simulink model "PPS_EGO_State_Display"  (Simulink 7.6)
settings: Solver=FixedStepDiscrete  SolverMode=SingleTasking  StartTime=0.0  StopTime=inf  FixedStep=0.01  RelTol=1e-3
InitFcn:
  | global det_flag;
  | 
  | det_flag = 0;
libraries: simulink x1
settings Model: Creator=Krzysztof  LastModifiedBy=pastora
settings DataIOCC: LimitDataPoints=off  MaxDataPoints=1  SaveOutput=off  DSMLogging=off  InspectSignalLogs=on
settings OptimizationCC: InlineParams=on
settings DebuggingCC: UnknownTsInhSupMsg=none
settings ModelReferenceCC: ModelReferenceNumInstancesAllowed=Single

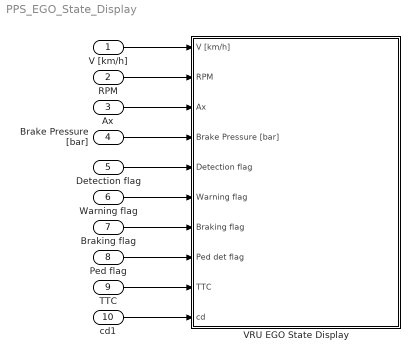
== system PPS_EGO_State_Display ==
  V [km/h] : Inport
  RPM : Inport  Port=2
  Ax : Inport  Port=3
  Brake Pressure [bar] : Inport  Port=4
  Detection flag : Inport  Port=5
  Warning flag : Inport  Port=6
  Braking flag : Inport  Port=7
  Ped flag : Inport  Port=8
  TTC : Inport  Port=9
  cd1 : Inport  Port=10
  VRU EGO State Display : Subsystem  mask{brakepressure=150, mfreq=100, dfreq=25}
      mask prompts: brakepressure "Maximum value of braking pressure [bar]"; mfreq "Model frequency [Hz]"; dfreq "Display frequency [Hz]"
  wires:
  V [km/h]/1 -> VRU EGO State Display/1(V [km/h])
  RPM/1 -> VRU EGO State Display/2(RPM)
  Brake Pressure [bar]/1 -> VRU EGO State Display/4(Brake Pressure [bar])
  Warning flag/1 -> VRU EGO State Display/6(Warning flag)
  Braking flag/1 -> VRU EGO State Display/7(Braking flag)
  Ped flag/1 -> VRU EGO State Display/8(Ped det flag)
  TTC/1 -> VRU EGO State Display/9(TTC)
  Detection flag/1 -> VRU EGO State Display/5(Detection flag)
  cd1/1 -> VRU EGO State Display/10(cd)
  Ax/1 -> VRU EGO State Display/3(Ax)

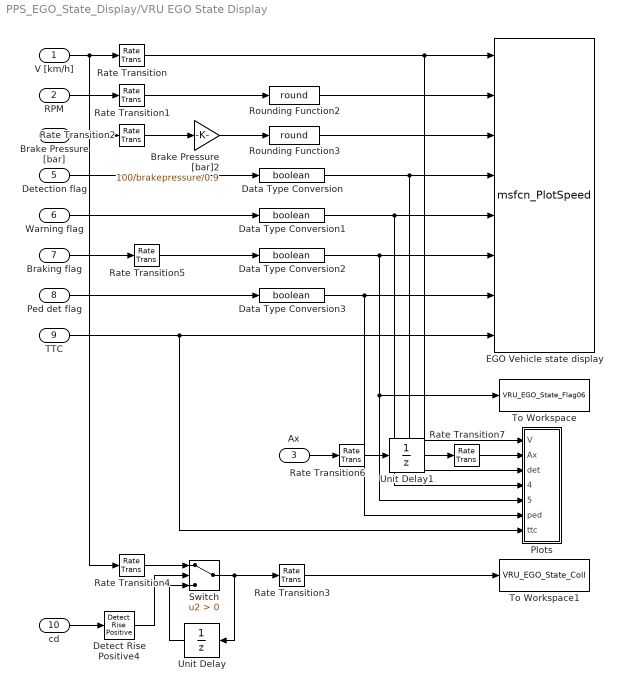
== system PPS_EGO_State_Display/VRU EGO State Display ==
  V [km/h] : Inport  SampleTime=[0,0]
  RPM : Inport  Port=2  SampleTime=[0,0]
  Ax : Inport  Port=3  SampleTime=[0,0]
  Brake Pressure [bar] : Inport  Port=4  SampleTime=[0,0]
  Detection flag : Inport  Port=5  OutDataTypeStr=boolean
  Warning flag : Inport  Port=6  OutDataTypeStr=boolean
  Braking flag : Inport  Port=7  OutDataTypeStr=boolean
  Ped det flag : Inport  Port=8  OutDataTypeStr=boolean
  TTC : Inport  Port=9  SampleTime=1/dfreq
  cd : Inport  Port=10  OutDataTypeStr=boolean  SampleTime=1/mfreq
  Brake Pressure [bar]2 : Gain  Gain=100/brakepressure/0.9
  Data Type Conversion{,1..3} (4 alike) : DataTypeConversion  OutDataTypeStr=boolean
  Detect Rise Positive4 : simulink/Logic and Bit Operations/Detect Rise Positive  SystemSampleTime=-1  vinit=0
  EGO Vehicle state display : M-S-Function  StopFcn=|  FunctionName=msfcn_PlotSpeed  Parameters=dfreq
      | CSpanel = findobj('Tag','cs_panel');                                                                                          
      | CSvalue = findobj('Tag','cs_value');                                                                                          
      | if VRU_EGO_State_Coll                                                                                                         
      |    % Collision occured                                                                                                        
      |    set(CSpanel, 'BorderWidth',2, 'ForegroundColor','Red', 'HighlightColor','Red', 'ShadowColor', 'Red');                      
      |    set(CSvalue, 'ForegroundColor','Red', 'String', strcat('Collision speed', sprintf( ' %.1f ',VRU_EGO_State_Coll), ' km/h'));
      |    set(CSpanel, 'Visible', 'On');                                                                                             
      |    set(CSvalue, 'Visible', 'On');                                                                                             
      | else                                                                                                                          
      |     if VRU_EGO_State_Flag06                                                                                                   
      |         % Collision almost occur                                                                                              
      | 	set(CSpanel, 'BorderWidth',2, 'ForegroundColor','Green', 'HighlightColor','Green', 'ShadowColor', 'Green');                  
      | 	set(CSvalue, 'ForegroundColor','Green', 'String', 'Collision avoided');                                                      
      |         set(CSpanel, 'Visible', 'On');                                                                                        
      |         set(CSvalue, 'Visible', 'On');                                                                                        
      |     else                                                                                                                      
      |         % No risk of collision                                                                                                
      | 	set(CSpanel, 'Visible', 'Off');                                                                                              
      |         set(CSvalue, 'Visible', 'Off');                                                                                       
      |     end                                                                                                                       
      | end                                                                                                                           
      | clear CSpanel CSvalue VRU_EGO_State_Flag06
  Plots : Subsystem  StopFcn=|
      | VRU_Speed_Profile(VRU_simout,VRU_EGO_State_Coll);
      | VRU_TTC_Profile(VRU_simout,VRU_EGO_State_Coll);
      mask Description:
      | The block calls functions:
      | * VRU_Speed_Profile
      | * VRU_TTC_Profile
      | to generate plots at the end of the simulation.
      | See stop callback of the block for more details.
  Rate Transition{,1..2,5,7} (5 alike) : RateTransition  Integrity=off  OutPortSampleTime=1/dfreq
  Rate Transition3 : RateTransition  Integrity=off  OutPortSampleTime=[0,0]
  Rate Transition4 : RateTransition  Integrity=off  OutPortSampleTime=1/mfreq
  Rate Transition6 : RateTransition  Integrity=off  OutPortSampleTimeOpt=Inherit  OutPortSampleTime=1/dfreq
  Rounding Function2 : Rounding  Operator=round
  Rounding Function3 : Rounding  Operator=round
  Switch : Switch  Criteria=u2 > Threshold  SampleTime=1/mfreq
  To Workspace : ToWorkspace  VariableName=VRU_EGO_State_Flag06  SampleTime=-1  SaveFormat=Array
      settings: MaxDataPoints=1
  To Workspace1 : ToWorkspace  VariableName=VRU_EGO_State_Coll  SampleTime=-1  SaveFormat=Array
      settings: MaxDataPoints=1
  Unit Delay : UnitDelay  SampleTime=1/mfreq
  Unit Delay1 : UnitDelay  SampleTime=-1
  wires:
  RPM/1 -> Rate Transition1/1
  Brake Pressure [bar]/1 -> Rate Transition2/1
  V [km/h]/1 -> Rate Transition/1, Rate Transition4/1
  Rounding Function2/1 -> EGO Vehicle state display/2
  Rounding Function3/1 -> EGO Vehicle state display/3
  Brake Pressure [bar]2/1 -> Rounding Function3/1
  Warning flag/1 -> Data Type Conversion1/1
  Ped det flag/1 -> Data Type Conversion3/1
  TTC/1 -> EGO Vehicle state display/8, Plots/7(ttc)
  Detection flag/1 -> Data Type Conversion/1
  Data Type Conversion/1 -> EGO Vehicle state display/4, Plots/3(det)
  Data Type Conversion1/1 -> EGO Vehicle state display/5, Plots/4(warn)
  Data Type Conversion2/1 -> EGO Vehicle state display/6, To Workspace/1, Plots/5(brake)
  Data Type Conversion3/1 -> EGO Vehicle state display/7, Plots/6(ped)
  Rate Transition/1 -> EGO Vehicle state display/1, Plots/1(V)
  Rate Transition1/1 -> Rounding Function2/1
  Rate Transition3/1 -> To Workspace1/1
  cd/1 -> Detect Rise Positive4/1
  Switch/1 -> Unit Delay/1, Rate Transition3/1
  Unit Delay/1 -> Switch/3
  Rate Transition4/1 -> Switch/1
  Detect Rise Positive4/1 -> Switch/2
  Braking flag/1 -> Rate Transition5/1
  Rate Transition5/1 -> Data Type Conversion2/1
  Ax/1 -> Rate Transition6/1
  Unit Delay1/1 -> Rate Transition7/1
  Rate Transition6/1 -> Unit Delay1/1
  Rate Transition2/1 -> Brake Pressure [bar]2/1
  Rate Transition7/1 -> Plots/2(Ax)

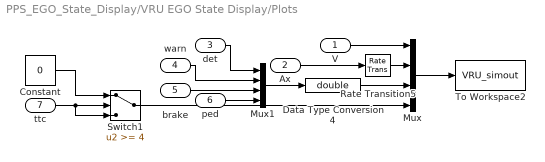
== system PPS_EGO_State_Display/VRU EGO State Display/Plots ==
  V : Inport
  Ax : Inport  Port=2  SampleTime=[0,0]
  det : Inport  Port=3
  warn : Inport  Port=4
  brake : Inport  Port=5
  ped : Inport  Port=6
  ttc : Inport  Port=7
  Constant : Constant  Value=0
  Data Type Conversion4 : DataTypeConversion  OutDataTypeStr=double
  Mux : Mux
  Mux1 : Mux
  Rate Transition5 : RateTransition  Integrity=off  OutPortSampleTime=1/dfreq
  Switch1 : Switch  Threshold=4
  To Workspace2 : ToWorkspace  VariableName=VRU_simout  SampleTime=0.04  SaveFormat=Structure With Time
  wires:
  Mux/1 -> To Workspace2/1
  Mux1/1 -> Data Type Conversion4/1
  Data Type Conversion4/1 -> Mux/3
  Ax/1 -> Rate Transition5/1
  Rate Transition5/1 -> Mux/2
  Switch1/1 -> Mux/4
  Constant/1 -> Switch1/1
  V/1 -> Mux/1
  det/1 -> Mux1/1
  warn/1 -> Mux1/2
  brake/1 -> Mux1/3
  ped/1 -> Mux1/4
  ttc/1 -> Switch1/2, Switch1/3
